simulink model "pid_model"  (Simulink 8.5)
settings: Solver=ode45  SolverMode=SingleTasking  StartTime=0.0  StopTime=15  RelTol=1e-3
values from neighbouring files (symbols this model uses):
  G_Denominator = str2double(get(hObject, 'String'))    [gui.m]    (also in variables.mat = [1 -4 3])
  G_Numerator = str2double(get(hObject, 'String'))    [gui.m]    (also in variables.mat = 1)
  H_Denominator = str2double(get(hObject, 'String'))    [gui.m]    (also in variables.mat = 1)
  H_Numerator = str2double(get(hObject, 'String'))    [gui.m]    (also in variables.mat = 1)
  observation_time = 10    [variables.mat]
  PID_D = str2double(get(hObject, 'String'))    [gui.m]    (also in variables.mat = 1000)
  PID_I = str2double(get(hObject, 'String'))    [gui.m]    (also in variables.mat = 0)
  PID_P = str2double(get(hObject, 'String'))    [gui.m]    (also in variables.mat = 17500)
  settling_time = 0.027    [variables.mat]
libraries: simulink x2, vrlib x1
settings Model: Creator=arekmano  LastModifiedBy=arekm  CovMetricSettings=dwe  CovHtmlReporting=off  covSaveCumulativeToWorkspaceVar=off  CovSaveSingleToWorkspaceVar=off  CovExternalEMLEnable=on
settings DataIOCC: LimitDataPoints=off  SaveFormat=Dataset  SignalLoggingSaveFormat=Dataset
settings OptimizationCC: ExpressionDepthLimit=128
settings DebuggingCC: UnderspecifiedInitializationDetection=Simplified  MergeDetectMultiDrivingBlocksExec=error  FcnCallInpInsideContextMsg=EnableAllAsError  StateNameClashWarn=none  SFUnexpectedBacktrackingDiag=error  SFNoUnconditionalDefaultTransitionDiag=error
settings HardwareCC: ProdBitPerPointer=64  ProdLargestAtomicFloat=Float  ProdIntDivRoundTo=Zero  ProdEndianess=LittleEndian  ProdHWDeviceType=Specified
settings ModelReferenceCC: PropagateSignalLabelsOutOfModel=on
settings GRTTargetCC: TargetLangStandard=C99 (ISO)  GeneratePreprocessorConditionals=Use local settings  CombineOutputUpdateFcns=on  GRTInterface=off

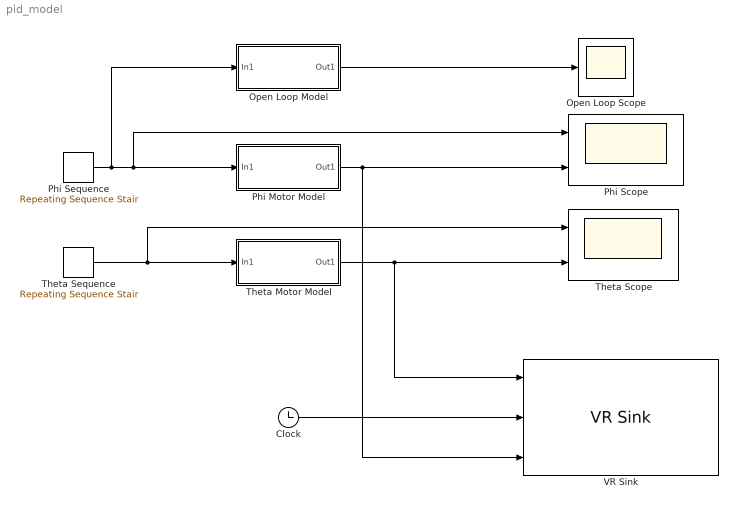
== system pid_model ==
  Clock : Clock
  Open Loop Model : Subsystem
  Open Loop Scope : Scope
      settings: SaveName=ScopeData2
  Phi Motor Model : Subsystem
  Phi Scope : Scope  NumInputPorts=2
      settings: ShowLegends=on  YMin=-2.31225~-5  YMax=20.81028~5
  Phi Sequence : simulink/Sources/Repeating Sequence Stair  OutValues=phi_inputs  tsamp=settling_time + observation_time  OutMin=[]  OutMax=[]  OutDataTypeStr=double  OutputDataTypeScalingMode=double  OutDataType=fixdt(0,8)  ConRadixGroup=Best Precision: Vector-wise  OutScaling=2^-12
  Theta Motor Model : Subsystem
  Theta Scope : Scope  NumInputPorts=2
      settings: ShowLegends=on  YMin=-33.39921~-5  YMax=300.59293~5
  Theta Sequence : simulink/Sources/Repeating Sequence Stair  OutValues=theta_inputs  tsamp=settling_time + observation_time  OutMin=[]  OutMax=[]  OutDataTypeStr=double  OutputDataTypeScalingMode=double  OutDataType=fixdt(0,8)  ConRadixGroup=Best Precision: Vector-wise  OutScaling=2^-12
  VR Sink : vrlib/VR Sink  InstantiateOnLoad=on  SampleTime=0.1  ViewEnable=on  RemoteChange=off  RemoteView=off  FieldsWritten=cyl_theta.height.1.1.1.double#cyl_time.height.1.1.1.double#cyl_phi.height.1.1.1.double  WorldFileName=vr_animation.wrl  AutoView=off  VideoDimensions=[]  AllowVariableSize=off
  wires:
  Phi Motor Model/1(Out1) -> Phi Scope/2, VR Sink/3
  Phi Sequence/1 -> Open Loop Model/1(In1), Phi Scope/1, Phi Motor Model/1(In1)
  Theta Sequence/1 -> Theta Scope/1, Theta Motor Model/1(In1)
  Theta Motor Model/1(Out1) -> VR Sink/1, Theta Scope/2
  Clock/1 -> VR Sink/2
  Open Loop Model/1(Out1) -> Open Loop Scope/1

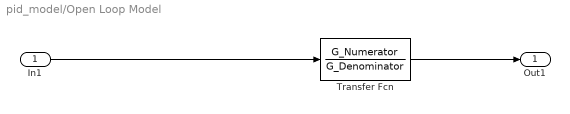
== system pid_model/Open Loop Model ==
  In1 : Inport
  Transfer Fcn : TransferFcn  Numerator=G_Numerator  Denominator=G_Denominator
  Out1 : Outport
  wires:
  Transfer Fcn/1 -> Out1/1
  In1/1 -> Transfer Fcn/1

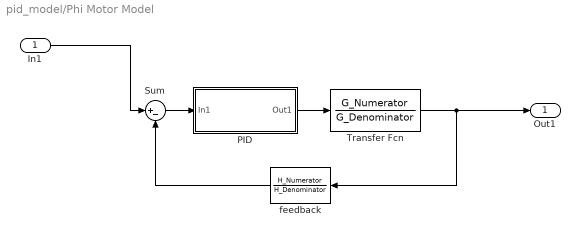
== system pid_model/Phi Motor Model ==
  In1 : Inport
  PID : Subsystem
  Sum : Sum  Inputs=|+-
  Transfer Fcn : TransferFcn  Numerator=G_Numerator  Denominator=G_Denominator
  feedback : TransferFcn  Numerator=H_Numerator  Denominator=H_Denominator
  Out1 : Outport
  wires:
  In1/1 -> Sum/1
  PID/1(Out1) -> Transfer Fcn/1
  Transfer Fcn/1 -> feedback/1, Out1/1
  feedback/1 -> Sum/2
  Sum/1 -> PID/1(In1)

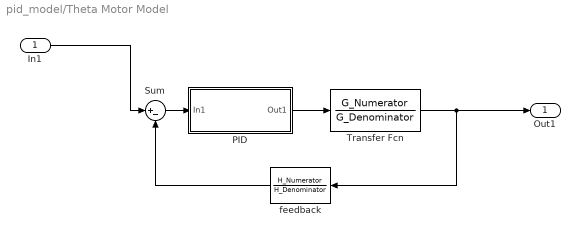
== system pid_model/Theta Motor Model ==
  In1 : Inport
  PID : Subsystem
  Sum : Sum  Inputs=|+-
  Transfer Fcn : TransferFcn  Numerator=G_Numerator  Denominator=G_Denominator
  feedback : TransferFcn  Numerator=H_Numerator  Denominator=H_Denominator
  Out1 : Outport
  wires:
  In1/1 -> Sum/1
  PID/1(Out1) -> Transfer Fcn/1
  Transfer Fcn/1 -> feedback/1, Out1/1
  Sum/1 -> PID/1(In1)
  feedback/1 -> Sum/2

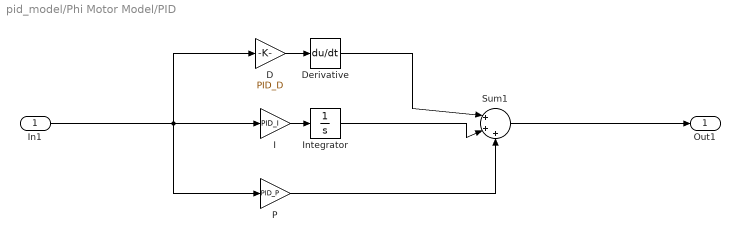
== system pid_model/Phi Motor Model/PID ==
  In1 : Inport
  D : Gain  Gain=PID_D
  Derivative : Derivative
  I : Gain  Gain=PID_I
  Integrator : Integrator
  P : Gain  Gain=PID_P
  Sum1 : Sum  Inputs=|+++
  Out1 : Outport
  wires:
  In1/1 -> P/1, I/1, D/1
  D/1 -> Derivative/1
  I/1 -> Integrator/1
  Integrator/1 -> Sum1/2
  P/1 -> Sum1/3
  Derivative/1 -> Sum1/1
  Sum1/1 -> Out1/1

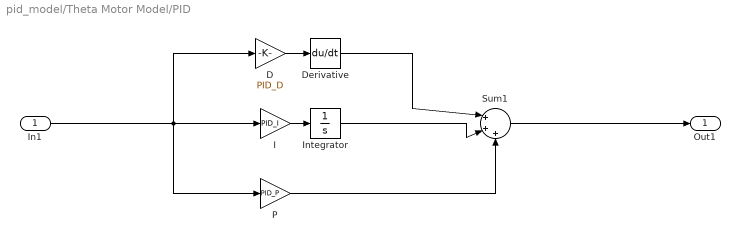
== system pid_model/Theta Motor Model/PID ==
  In1 : Inport
  D : Gain  Gain=PID_D
  Derivative : Derivative
  I : Gain  Gain=PID_I
  Integrator : Integrator
  P : Gain  Gain=PID_P
  Sum1 : Sum  Inputs=|+++
  Out1 : Outport
  wires:
  In1/1 -> P/1, I/1, D/1
  D/1 -> Derivative/1
  I/1 -> Integrator/1
  Integrator/1 -> Sum1/2
  P/1 -> Sum1/3
  Derivative/1 -> Sum1/1
  Sum1/1 -> Out1/1
